simulink library "UAVdesign_net"  (Simulink 7.7)
settings: Solver=ode45  SolverMode=SingleTasking  StartTime=0.0  StopTime=10.0  RelTol=1e-3
undefined symbols (not defined in the file or in its folder): alpha_IERA_IELA_IELA, R_IERA_RA_RA
libraries: UAVdesign_net x75, simulink x13
(part 6 of 8)

== system UAVdesign_net/Subsystem Models/Helicopter Rotor/Rotor Model (IERA)/Rotor Flapping ==
  Parameters : Inport  OutDataTypeStr=Bus: RotorParameters
  Environment : Inport  Port=2  OutDataTypeStr=Bus: Environment
  V_I : Inport  Port=3
  omega_I : Inport  Port=4
  V_dot_I : Inport  Port=5
  omega_dot_I : Inport  Port=6
  V_A : Inport  Port=7
  omega_A : Inport  Port=8
  flap : Inport  Port=9
  cz : Inport  Port=10
  controls : Inport  Port=11
  omega : Inport  Port=12
  Rotor Flapping (Wind-Mast axes) : Stateflow chart  TreatAsAtomicUnit=on
  flap_dot : Outport  PortDimensions=3
  flap_static : Outport  Port=2  PortDimensions=3
  wires:
  Rotor Flapping (Wind-Mast axes)/2(flap_static) -> flap_static/1
  Rotor Flapping (Wind-Mast axes)/1(flap_dot) -> flap_dot/1
  omega/1 -> Rotor Flapping (Wind-Mast axes)/12(omega)
  controls/1 -> Rotor Flapping (Wind-Mast axes)/11(controls)
  cz/1 -> Rotor Flapping (Wind-Mast axes)/10(cz)
  flap/1 -> Rotor Flapping (Wind-Mast axes)/9(flap)
  omega_A/1 -> Rotor Flapping (Wind-Mast axes)/8(oma)
  V_A/1 -> Rotor Flapping (Wind-Mast axes)/7(va)
  omega_dot_I/1 -> Rotor Flapping (Wind-Mast axes)/6(omid)
  V_dot_I/1 -> Rotor Flapping (Wind-Mast axes)/5(vid)
  omega_I/1 -> Rotor Flapping (Wind-Mast axes)/4(omi)
  V_I/1 -> Rotor Flapping (Wind-Mast axes)/3(vi)
  Environment/1 -> Rotor Flapping (Wind-Mast axes)/2(Environment)
  Parameters/1 -> Rotor Flapping (Wind-Mast axes)/1(Parameters)

== system UAVdesign_net/Subsystem Models/Helicopter Rotor/Rotor Model (IERA)/Rotor Forces and Moments ==
  Parameters : Inport  OutDataTypeStr=Bus: RotorParameters
  Environment : Inport  Port=2  OutDataTypeStr=Bus: Environment
  V_A : Inport  Port=3
  omega_A : Inport  Port=4
  omega_dot_I : Inport  Port=5
  flap : Inport  Port=6
  cz : Inport  Port=7
  controls : Inport  Port=8
  omega_rotor : Inport  Port=9
  omega_dot_rotor : Inport  Port=10
  Rotor Forces and Moments (Wind-Mast axes) : Stateflow chart  TreatAsAtomicUnit=on
  FM_A : Outport  PortDimensions=6
  FM_I : Outport  Port=2  PortDimensions=6
  wires:
  Rotor Forces and Moments (Wind-Mast axes)/2(FM_I) -> FM_I/1
  Rotor Forces and Moments (Wind-Mast axes)/1(FM_A) -> FM_A/1
  omega_dot_rotor/1 -> Rotor Forces and Moments (Wind-Mast axes)/10(omegad)
  omega_rotor/1 -> Rotor Forces and Moments (Wind-Mast axes)/9(omega)
  controls/1 -> Rotor Forces and Moments (Wind-Mast axes)/8(controls)
  cz/1 -> Rotor Forces and Moments (Wind-Mast axes)/7(cz)
  flap/1 -> Rotor Forces and Moments (Wind-Mast axes)/6(flap)
  omega_dot_I/1 -> Rotor Forces and Moments (Wind-Mast axes)/5(omid)
  omega_A/1 -> Rotor Forces and Moments (Wind-Mast axes)/4(oma)
  V_A/1 -> Rotor Forces and Moments (Wind-Mast axes)/3(va)
  Environment/1 -> Rotor Forces and Moments (Wind-Mast axes)/2(Environment)
  Parameters/1 -> Rotor Forces and Moments (Wind-Mast axes)/1(Parameters)

== system UAVdesign_net/Subsystem Models/Helicopter Rotor/Rotor Model (IERA)/Rotor Self-Influence ==
  Parameters : Inport  OutDataTypeStr=Bus: RotorParameters
  Environment : Inport  Port=2  OutDataTypeStr=Bus: Environment
  V_A : Inport  Port=3
  omega_A : Inport  Port=4
  FM_A : Inport  Port=5
  Rotor Wash Self-Influence (IERA) : Stateflow chart  TreatAsAtomicUnit=on
  d (k) : Outport  PortDimensions=3
  wires:
  Parameters/1 -> Rotor Wash Self-Influence (IERA)/1(Parameters)
  Rotor Wash Self-Influence (IERA)/1(d) -> d (k)/1
  Environment/1 -> Rotor Wash Self-Influence (IERA)/2(Environment)
  V_A/1 -> Rotor Wash Self-Influence (IERA)/3(va)
  omega_A/1 -> Rotor Wash Self-Influence (IERA)/4(oma)
  FM_A/1 -> Rotor Wash Self-Influence (IERA)/5(FM_A)

== system UAVdesign_net/Subsystem Models/Helicopter Rotor/Rotor Model (IERA)/Rotor Wash Iteration ==
  Parameters : Inport  OutDataTypeStr=Bus: RotorParameters
  V_I : Inport  Port=2
  V_A (k-1) : Inport  Port=3
  omega_A : Inport  Port=4
  bt (k-1) : Inport  Port=5
  eps0 (k-1) : Inport  Port=6
  controls : Inport  Port=7
  omega_rotor : Inport  Port=8
  Rotor Wash Iteration (Wind-Mast axes) : Stateflow chart  TreatAsAtomicUnit=on
  V_A (k) : Outport  PortDimensions=3
  cz (k) : Outport  Port=2  PortDimensions=1
  bt (k) : Outport  Port=3  PortDimensions=1
  eps0 (k) : Outport  Port=4  PortDimensions=1
  wires:
  omega_rotor/1 -> Rotor Wash Iteration (Wind-Mast axes)/8(omega)
  controls/1 -> Rotor Wash Iteration (Wind-Mast axes)/7(controls)
  eps0 (k-1)/1 -> Rotor Wash Iteration (Wind-Mast axes)/6(eps0)
  bt (k-1)/1 -> Rotor Wash Iteration (Wind-Mast axes)/5(bt)
  omega_A/1 -> Rotor Wash Iteration (Wind-Mast axes)/4(oma)
  V_A (k-1)/1 -> Rotor Wash Iteration (Wind-Mast axes)/3(va)
  V_I/1 -> Rotor Wash Iteration (Wind-Mast axes)/2(vi)
  Rotor Wash Iteration (Wind-Mast axes)/4(eps0_new) -> eps0 (k)/1
  Rotor Wash Iteration (Wind-Mast axes)/3(bt_new) -> bt (k)/1
  Rotor Wash Iteration (Wind-Mast axes)/2(cz_new) -> cz (k)/1
  Rotor Wash Iteration (Wind-Mast axes)/1(va_new) -> V_A (k)/1
  Parameters/1 -> Rotor Wash Iteration (Wind-Mast axes)/1(Parameters)

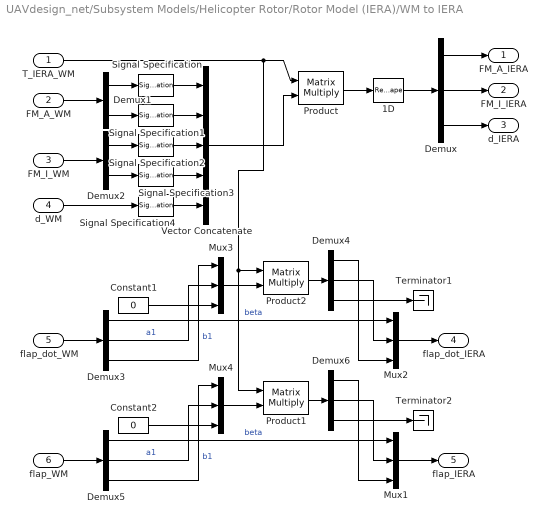
== system UAVdesign_net/Subsystem Models/Helicopter Rotor/Rotor Model (IERA)/WM to IERA ==
  T_IERA_WM : Inport
  FM_A_WM : Inport  Port=2  PortDimensions=6
  FM_I_WM : Inport  Port=3  PortDimensions=6
  d_WM : Inport  Port=4  PortDimensions=3
  flap_dot_WM : Inport  Port=5
  flap_WM : Inport  Port=6
  1D : Reshape
  Constant1 : Constant  Value=0
  Constant2 : Constant  Value=0
  Demux : Demux  Outputs=[6 6 3]
  Demux1 : Demux  Outputs=[3 3]
  Demux2 : Demux  Outputs=[3 3]
  Demux{3..6} (4 alike) : Demux  Outputs=3
  Mux{1..4} (4 alike) : Mux  Inputs=3
  Product : Product  Multiplication=Matrix(*)  RndMeth=Zero
  Product1 : Product  Multiplication=Matrix(*)  RndMeth=Zero
  Product2 : Product  Multiplication=Matrix(*)  RndMeth=Zero
  Signal Specification{,1..4} (5 alike) : SignalSpecification  Dimensions=3
  Terminator1 : Terminator
  Terminator2 : Terminator
  Vector Concatenate : Concatenate  NumInputs=5  Mode=Multidimensional array  ConcatenateDimension=2
  FM_A_IERA : Outport
  FM_I_IERA : Outport  Port=2
  d_IERA : Outport  Port=3
  flap_dot_IERA : Outport  Port=4
  flap_IERA : Outport  Port=5
  wires:
  flap_WM/1 -> Demux5/1
  Mux1/1 -> flap_IERA/1
  Demux5/1 -> Mux1/1  "beta"
  Demux5/2 -> Mux4/2  "a1"
  Demux5/3 -> Mux4/1  "b1"
  Constant2/1 -> Mux4/3
  Mux4/1 -> Product1/2
  Product1/1 -> Demux6/1
  Demux6/1 -> Mux1/3
  Demux6/2 -> Mux1/2
  Demux6/3 -> Terminator2/1
  Demux/2 -> FM_I_IERA/1
  Demux/3 -> d_IERA/1
  FM_I_WM/1 -> Demux2/1
  Demux2/2 -> Signal Specification3/1
  Demux2/1 -> Signal Specification2/1
  d_WM/1 -> Signal Specification4/1
  Demux/1 -> FM_A_IERA/1
  FM_A_WM/1 -> Demux1/1
  Demux1/2 -> Signal Specification1/1
  Demux1/1 -> Signal Specification/1
  1D/1 -> Demux/1
  Product/1 -> 1D/1
  Vector Concatenate/1 -> Product/2
  T_IERA_WM/1 -> Product1/1, Product2/1, Product/1
  flap_dot_WM/1 -> Demux3/1
  Mux2/1 -> flap_dot_IERA/1
  Demux3/1 -> Mux2/1  "beta"
  Demux3/2 -> Mux3/2  "a1"
  Demux3/3 -> Mux3/1  "b1"
  Constant1/1 -> Mux3/3
  Mux3/1 -> Product2/2
  Product2/1 -> Demux4/1
  Demux4/1 -> Mux2/3
  Demux4/2 -> Mux2/2
  Demux4/3 -> Terminator1/1
  Signal Specification/1 -> Vector Concatenate/1
  Signal Specification1/1 -> Vector Concatenate/2
  Signal Specification2/1 -> Vector Concatenate/3
  Signal Specification3/1 -> Vector Concatenate/4
  Signal Specification4/1 -> Vector Concatenate/5

== system UAVdesign_net/Subsystem Models/Helicopter Rotor/Rotor Model (IERA)/Wind-Mast Orientation ==
  V_A : Inport
  Wind Reference Axes : Stateflow chart  TreatAsAtomicUnit=on
  T_WM_IERA : Outport
  T_IERA_WM : Outport  Port=2
  wires:
  V_A/1 -> Wind Reference Axes/1(VA_IERA)
  Wind Reference Axes/1(T_WM_IERA) -> T_WM_IERA/1
  Wind Reference Axes/2(T_IERA_WM) -> T_IERA_WM/1

== system UAVdesign_net/Subsystem Models/Propeller/Rotor Model (IERA)/IERA to WM ==
  T_WM_IERA : Inport
  V_I_IERA : Inport  Port=2
  omega_I_IERA : Inport  Port=3
  V_A_IERA : Inport  Port=4
  omega_A_IERA : Inport  Port=5
  1D : Reshape
  Demux : Demux
  Product : Product  Multiplication=Matrix(*)  RndMeth=Zero
  Vector Concatenate : Concatenate  NumInputs=4  Mode=Multidimensional array  ConcatenateDimension=2
  V_I_WM : Outport
  omega_I_WM : Outport  Port=2
  V_A_WM : Outport  Port=3
  omega_A_WM : Outport  Port=4
  wires:
  Demux/2 -> omega_I_WM/1
  Demux/1 -> V_I_WM/1
  1D/1 -> Demux/1
  Product/1 -> 1D/1
  Vector Concatenate/1 -> Product/2
  omega_I_IERA/1 -> Vector Concatenate/2
  V_I_IERA/1 -> Vector Concatenate/1
  T_WM_IERA/1 -> Product/1
  V_A_IERA/1 -> Vector Concatenate/3
  omega_A_IERA/1 -> Vector Concatenate/4
  Demux/3 -> V_A_WM/1
  Demux/4 -> omega_A_WM/1

== system UAVdesign_net/Subsystem Models/Propeller/Rotor Model (IERA)/Rotor Forces and Moments (Aero) ==
  Parameters : Inport
  Environment : Inport  Port=2
  V_A : Inport  Port=3
  omega_A : Inport  Port=4
  cz : Inport  Port=5
  controls : Inport  Port=6
  omega_rotor : Inport  Port=7
  Rotor Forces and Moments (Wind-Mast axes) : Stateflow chart  TreatAsAtomicUnit=on
  FM_A : Outport  PortDimensions=6
  wires:
  Parameters/1 -> Rotor Forces and Moments (Wind-Mast axes)/1(Parameters)
  Environment/1 -> Rotor Forces and Moments (Wind-Mast axes)/2(Environment)
  V_A/1 -> Rotor Forces and Moments (Wind-Mast axes)/3(va)
  omega_A/1 -> Rotor Forces and Moments (Wind-Mast axes)/4(oma)
  cz/1 -> Rotor Forces and Moments (Wind-Mast axes)/5(cz)
  controls/1 -> Rotor Forces and Moments (Wind-Mast axes)/6(controls)
  omega_rotor/1 -> Rotor Forces and Moments (Wind-Mast axes)/7(omega)
  Rotor Forces and Moments (Wind-Mast axes)/1(FM_A) -> FM_A/1

== system UAVdesign_net/Subsystem Models/Propeller/Rotor Model (IERA)/Rotor Self-Influence ==
  Parameters : Inport
  Environment : Inport  Port=2
  V_A : Inport  Port=3
  omega_A : Inport  Port=4
  FM_A : Inport  Port=5
  Rotor Wash Self-Influence (IERA) : Stateflow chart  TreatAsAtomicUnit=on
  d (k) : Outport  PortDimensions=3
  wires:
  FM_A/1 -> Rotor Wash Self-Influence (IERA)/5(FM_A)
  omega_A/1 -> Rotor Wash Self-Influence (IERA)/4(oma)
  V_A/1 -> Rotor Wash Self-Influence (IERA)/3(va)
  Environment/1 -> Rotor Wash Self-Influence (IERA)/2(Environment)
  Rotor Wash Self-Influence (IERA)/1(d) -> d (k)/1
  Parameters/1 -> Rotor Wash Self-Influence (IERA)/1(Parameters)

== system UAVdesign_net/Subsystem Models/Propeller/Rotor Model (IERA)/Rotor Wash Iteration ==
  Parameters : Inport
  V_I : Inport  Port=2
  V_A (k-1) : Inport  Port=3
  omega_A : Inport  Port=4
  bt (k-1) : Inport  Port=5
  eps0 (k-1) : Inport  Port=6
  controls : Inport  Port=7
  omega_rotor : Inport  Port=8
  Rotor Wash Iteration (Wind-Mast axes) : Stateflow chart  TreatAsAtomicUnit=on
  V_A (k) : Outport  PortDimensions=3
  cz (k) : Outport  Port=2  PortDimensions=1
  bt (k) : Outport  Port=3  PortDimensions=1
  eps0 (k) : Outport  Port=4  PortDimensions=1
  wires:
  Parameters/1 -> Rotor Wash Iteration (Wind-Mast axes)/1(Parameters)
  Rotor Wash Iteration (Wind-Mast axes)/1(va_new) -> V_A (k)/1
  Rotor Wash Iteration (Wind-Mast axes)/2(cz_new) -> cz (k)/1
  Rotor Wash Iteration (Wind-Mast axes)/3(bt_new) -> bt (k)/1
  Rotor Wash Iteration (Wind-Mast axes)/4(eps0_new) -> eps0 (k)/1
  V_I/1 -> Rotor Wash Iteration (Wind-Mast axes)/2(vi)
  V_A (k-1)/1 -> Rotor Wash Iteration (Wind-Mast axes)/3(va)
  omega_A/1 -> Rotor Wash Iteration (Wind-Mast axes)/4(oma)
  bt (k-1)/1 -> Rotor Wash Iteration (Wind-Mast axes)/5(bt)
  eps0 (k-1)/1 -> Rotor Wash Iteration (Wind-Mast axes)/6(eps0)
  controls/1 -> Rotor Wash Iteration (Wind-Mast axes)/7(controls)
  omega_rotor/1 -> Rotor Wash Iteration (Wind-Mast axes)/8(omega)

== system UAVdesign_net/Subsystem Models/Propeller/Rotor Model (IERA)/WM to IERA ==
  T_IERA_WM : Inport
  FM_A_WM : Inport  Port=2  PortDimensions=6
  d_WM : Inport  Port=3  PortDimensions=3
  1D : Reshape
  Demux : Demux  Outputs=[6 3]
  Demux1 : Demux  Outputs=[3 3]
  Product : Product  Multiplication=Matrix(*)  RndMeth=Zero
  Signal Specification : SignalSpecification  Dimensions=3
  Signal Specification1 : SignalSpecification  Dimensions=3
  Signal Specification4 : SignalSpecification  Dimensions=3
  Vector Concatenate : Concatenate  NumInputs=3  Mode=Multidimensional array  ConcatenateDimension=2
  FM_A_IERA : Outport
  d_IERA : Outport  Port=2
  wires:
  Signal Specification4/1 -> Vector Concatenate/3
  Signal Specification1/1 -> Vector Concatenate/2
  Signal Specification/1 -> Vector Concatenate/1
  T_IERA_WM/1 -> Product/1
  Vector Concatenate/1 -> Product/2
  Product/1 -> 1D/1
  1D/1 -> Demux/1
  Demux1/1 -> Signal Specification/1
  Demux1/2 -> Signal Specification1/1
  FM_A_WM/1 -> Demux1/1
  Demux/1 -> FM_A_IERA/1
  d_WM/1 -> Signal Specification4/1
  Demux/2 -> d_IERA/1

== system UAVdesign_net/Subsystem Models/Propeller/Rotor Model (IERA)/Wind-Mast Orientation ==
  V_A : Inport
  Wind Reference Axes : Stateflow chart  TreatAsAtomicUnit=on
  T_WM_IERA : Outport
  T_IERA_WM : Outport  Port=2
  wires:
  Wind Reference Axes/2(T_IERA_WM) -> T_IERA_WM/1
  Wind Reference Axes/1(T_WM_IERA) -> T_WM_IERA/1
  V_A/1 -> Wind Reference Axes/1(VA_IERA)

== system UAVdesign_net/Subsystem Models/Wing/Wing Model (IERA)/Left Wing ==
  Parameters : Inport  OutDataTypeStr=Bus: FinParameters
  Environment : Inport  Port=2  OutDataTypeStr=Bus: Environment
  V_A : Inport  Port=3
  omega_A : Inport  Port=4
  T_WRA_MAC : Inport  Port=5
  T_MAC_WRA : Inport  Port=6
  Left/Right : Inport  Port=7
  Bus Selector : BusSelector  OutputSignals=taper,span,sweep,dihedral
  Half Wing Forces and Moments : Subsystem
      mask Display:
      | port_label('input', 1, 'Parameters', 'texmode', 'on')
      | port_label('input', 2, 'Environment', 'texmode', 'on')
      | port_label('input', 3, 'V_{A|WRA}', 'texmode', 'on')
      | port_label('input', 4, '\omega_{A|WRA}', 'texmode', 'on')
      | 
      | port_label('output', 1, 'FM_{A}', 'texmode', 'on')
  IERA to MAC : Subsystem
      mask Display:
      | port_label('input', 1, 'R_{MAC-IERA|IERA}', 'texmode', 'on')
      | port_label('input', 2, 'V_{A|IERA}', 'texmode', 'on')
      | port_label('input', 3, '\omega_{A|IERA}', 'texmode', 'on')
      | port_label('output', 1, 'V_{A|MAC}', 'texmode', 'on')
      | port_label('output', 2, '\omega_{A|MAC}', 'texmode', 'on')
  MAC to IERA : Subsystem
      mask Display:
      | port_label('input', 1, 'R_{MAC-IERA|IERA}', 'texmode', 'on')
      | port_label('input', 2, 'FM_{MAC}', 'texmode', 'on')
      | port_label('output', 1, 'FM_{IERA}', 'texmode', 'on')
  MAC to WRA (Half Wing) : Subsystem
      mask Display:
      | port_label('input', 1, 'T_{WRA-MAC}', 'texmode', 'on')
      | port_label('input', 2, 'V_{A|MAC}', 'texmode', 'on')
      | port_label('input', 3, '\omega_{A|MAC}', 'texmode', 'on')
      | 
      | port_label('output', 1, 'V_{A|WRA}', 'texmode', 'on')
      | port_label('output', 2, '\omega_{A|WRA}', 'texmode', 'on')
  Mux1 : Mux
  Mux2 : Mux  Inputs=2
  Mux3 : Mux  Inputs=3
  WRA to MAC : Subsystem
      mask Display:
      | port_label('input', 1, 'T_{MAC-WRA}', 'texmode', 'on')
      | port_label('input', 2, 'FM_{A|WRA}', 'texmode', 'on')
      | 
      | port_label('output', 1, 'FM_{A|MAC}', 'texmode', 'on')
  smac : Fcn  Expr=u(2) * (2 * u(1) + 1) / 6 / (u(1) + 1)
  xmac : Fcn  Expr=-sin(u(2)) * cos(-u(3)) * u(1)
  ymac : Fcn  Expr=u(4) * cos(u(2)) * cos(-u(3)) * u(1)
  zmac : Fcn  Expr=sin(-u(3)) * u(1)
  FM_A : Outport
  wires:
  Half Wing Forces and Moments/1(FM_A) -> WRA to MAC/2(FM_A_WM)
  IERA to MAC/1(V_A|MAC) -> MAC to WRA (Half Wing)/2(V_A_MAC)
  IERA to MAC/2(omega_A|MAC) -> MAC to WRA (Half Wing)/3(omega_A_MAC)
  zmac/1 -> Mux3/3
  ymac/1 -> Mux3/2
  xmac/1 -> Mux3/1
  Mux3/1 -> IERA to MAC/1(R_xW-IERA|IERA), MAC to IERA/1(R_MAC_IERA_IERA)
  MAC to WRA (Half Wing)/1(V_A_WRA) -> Half Wing Forces and Moments/3(V_A)
  MAC to WRA (Half Wing)/2(omega_A_WRA) -> Half Wing Forces and Moments/4(omega_A)
  Parameters/1 -> Half Wing Forces and Moments/1(Parameters), Bus Selector/1
  T_WRA_MAC/1 -> MAC to WRA (Half Wing)/1(T_WRA_MAC)
  T_MAC_WRA/1 -> WRA to MAC/1(T_IERA_WM)
  V_A/1 -> IERA to MAC/2(V_A|IERA)
  omega_A/1 -> IERA to MAC/3(omega_A|IERA)
  Mux1/1 -> ymac/1, xmac/1, zmac/1
  Left/Right/1 -> Mux1/4
  smac/1 -> Mux1/1
  Environment/1 -> Half Wing Forces and Moments/2(Environment)
  Bus Selector/1 -> Mux2/1  "<taper>"
  Bus Selector/2 -> Mux2/2  "<span>"
  Mux2/1 -> smac/1
  Bus Selector/3 -> Mux1/2  "<sweep>"
  Bus Selector/4 -> Mux1/3  "<dihedral>"
  WRA to MAC/1(FM_A_IERA) -> MAC to IERA/2(FM_MAC)
  MAC to IERA/1(FM_IERA) -> FM_A/1

== system UAVdesign_net/Subsystem Models/Wing/Wing Model (IERA)/Right Wing ==
  Parameters : Inport  OutDataTypeStr=Bus: FinParameters
  Environment : Inport  Port=2  OutDataTypeStr=Bus: Environment
  V_A : Inport  Port=3
  omega_A : Inport  Port=4
  T_WRA_MAC : Inport  Port=5
  T_MAC_WRA : Inport  Port=6
  Left/Right : Inport  Port=7
  Bus Selector : BusSelector  OutputSignals=taper,span,sweep,dihedral
  Half Wing Forces and Moments : Subsystem
      mask Display:
      | port_label('input', 1, 'Parameters', 'texmode', 'on')
      | port_label('input', 2, 'Environment', 'texmode', 'on')
      | port_label('input', 3, 'V_{A|WRA}', 'texmode', 'on')
      | port_label('input', 4, '\omega_{A|WRA}', 'texmode', 'on')
      | 
      | port_label('output', 1, 'FM_{A}', 'texmode', 'on')
  IERA to MAC : Subsystem
      mask Display:
      | port_label('input', 1, 'R_{MAC-IERA|IERA}', 'texmode', 'on')
      | port_label('input', 2, 'V_{A|IERA}', 'texmode', 'on')
      | port_label('input', 3, '\omega_{A|IERA}', 'texmode', 'on')
      | port_label('output', 1, 'V_{A|MAC}', 'texmode', 'on')
      | port_label('output', 2, '\omega_{A|MAC}', 'texmode', 'on')
  MAC to IERA : Subsystem
      mask Display:
      | port_label('input', 1, 'R_{MAC-IERA|IERA}', 'texmode', 'on')
      | port_label('input', 2, 'FM_{MAC}', 'texmode', 'on')
      | port_label('output', 1, 'FM_{IERA}', 'texmode', 'on')
  MAC to WRA (Half Wing) : Subsystem
      mask Display:
      | port_label('input', 1, 'T_{WRA-MAC}', 'texmode', 'on')
      | port_label('input', 2, 'V_{A|MAC}', 'texmode', 'on')
      | port_label('input', 3, '\omega_{A|MAC}', 'texmode', 'on')
      | 
      | port_label('output', 1, 'V_{A|WRA}', 'texmode', 'on')
      | port_label('output', 2, '\omega_{A|WRA}', 'texmode', 'on')
  Mux1 : Mux
  Mux2 : Mux  Inputs=2
  Mux3 : Mux  Inputs=3
  WRA to MAC : Subsystem
      mask Display:
      | port_label('input', 1, 'T_{MAC-WRA}', 'texmode', 'on')
      | port_label('input', 2, 'FM_{A|WRA}', 'texmode', 'on')
      | 
      | port_label('output', 1, 'FM_{A|MAC}', 'texmode', 'on')
  smac : Fcn  Expr=u(2) * (2 * u(1) + 1) / 6 / (u(1) + 1)
  xmac : Fcn  Expr=-sin(u(2)) * cos(-u(3)) * u(1)
  ymac : Fcn  Expr=u(4) * cos(u(2)) * cos(-u(3)) * u(1)
  zmac : Fcn  Expr=sin(-u(3)) * u(1)
  FM_A : Outport
  wires:
  MAC to IERA/1(FM_IERA) -> FM_A/1
  WRA to MAC/1(FM_A_IERA) -> MAC to IERA/2(FM_MAC)
  Bus Selector/4 -> Mux1/3  "<dihedral>"
  Bus Selector/3 -> Mux1/2  "<sweep>"
  Mux2/1 -> smac/1
  Bus Selector/2 -> Mux2/2  "<span>"
  Bus Selector/1 -> Mux2/1  "<taper>"
  Environment/1 -> Half Wing Forces and Moments/2(Environment)
  smac/1 -> Mux1/1
  Left/Right/1 -> Mux1/4
  Mux1/1 -> zmac/1, xmac/1, ymac/1
  omega_A/1 -> IERA to MAC/3(omega_A|IERA)
  V_A/1 -> IERA to MAC/2(V_A|IERA)
  T_MAC_WRA/1 -> WRA to MAC/1(T_IERA_WM)
  T_WRA_MAC/1 -> MAC to WRA (Half Wing)/1(T_WRA_MAC)
  Parameters/1 -> Bus Selector/1, Half Wing Forces and Moments/1(Parameters)
  MAC to WRA (Half Wing)/2(omega_A_WRA) -> Half Wing Forces and Moments/4(omega_A)
  MAC to WRA (Half Wing)/1(V_A_WRA) -> Half Wing Forces and Moments/3(V_A)
  Mux3/1 -> MAC to IERA/1(R_MAC_IERA_IERA), IERA to MAC/1(R_xW-IERA|IERA)
  xmac/1 -> Mux3/1
  ymac/1 -> Mux3/2
  zmac/1 -> Mux3/3
  IERA to MAC/2(omega_A|MAC) -> MAC to WRA (Half Wing)/3(omega_A_MAC)
  IERA to MAC/1(V_A|MAC) -> MAC to WRA (Half Wing)/2(V_A_MAC)
  Half Wing Forces and Moments/1(FM_A) -> WRA to MAC/2(FM_A_WM)

== system UAVdesign_net/Subsystem Models/Wing/Wing Model (IERA)/Transpose ==
  In : Inport
  Permute Dimensions : PermuteDimensions
  Out : Outport
  wires:
  In/1 -> Permute Dimensions/1
  Permute Dimensions/1 -> Out/1

== system UAVdesign_net/Subsystem Models/Wing/Wing Model (IERA)/Wing Self-Influence ==
  Parameters : Inport  OutDataTypeStr=Bus: FinParameters
  Environment : Inport  Port=2  OutDataTypeStr=Bus: Environment
  V_A : Inport  Port=3
  omega_A : Inport  Port=4
  FM_A : Inport  Port=5
  Wing Wash Self-Influence (IERA : Stateflow chart  TreatAsAtomicUnit=on
  d (k) : Outport
  wires:
  Parameters/1 -> Wing Wash Self-Influence (IERA/1(Parameters)
  Wing Wash Self-Influence (IERA/1(d) -> d (k)/1
  Environment/1 -> Wing Wash Self-Influence (IERA/2(Environment)
  V_A/1 -> Wing Wash Self-Influence (IERA/3(va)
  omega_A/1 -> Wing Wash Self-Influence (IERA/4(oma)
  FM_A/1 -> Wing Wash Self-Influence (IERA/5(FM_A)

== system UAVdesign_net/Utilities/Math/3x3 Cross Product/Subsystem ==
  A : Inport
  B : Inport  Port=2
  Demux : Demux  Outputs=3
  Demux1 : Demux  Outputs=3
  Mux : Mux  Inputs=3
  i x j : Product  SaturateOnIntegerOverflow=on  InputSameDT=on  OutDataTypeStr=Inherit: Same as first input
  j x k : Product  SaturateOnIntegerOverflow=on  InputSameDT=on  OutDataTypeStr=Inherit: Same as first input
  k x i : Product  SaturateOnIntegerOverflow=on  InputSameDT=on  OutDataTypeStr=Inherit: Same as first input
  Out1 : Outport
  wires:
  Mux/1 -> Out1/1
  A/1 -> Demux/1
  B/1 -> Demux1/1
  j x k/1 -> Mux/1
  k x i/1 -> Mux/2
  i x j/1 -> Mux/3
  Demux/1 -> i x j/1
  Demux1/2 -> i x j/2
  Demux1/1 -> k x i/2
  Demux/3 -> k x i/1
  Demux/2 -> j x k/1
  Demux1/3 -> j x k/2

== system UAVdesign_net/Utilities/Math/3x3 Cross Product/Subsystem1 ==
  A : Inport
  B : Inport  Port=2
  Demux : Demux  Outputs=3
  Demux1 : Demux  Outputs=3
  Mux : Mux  Inputs=3
  i x k : Product  SaturateOnIntegerOverflow=on  InputSameDT=on  OutDataTypeStr=Inherit: Same as first input
  j x i : Product  SaturateOnIntegerOverflow=on  InputSameDT=on  OutDataTypeStr=Inherit: Same as first input
  k x j : Product  SaturateOnIntegerOverflow=on  InputSameDT=on  OutDataTypeStr=Inherit: Same as first input
  Out1 : Outport
  wires:
  A/1 -> Demux/1
  B/1 -> Demux1/1
  Demux/3 -> k x j/1
  Demux1/2 -> k x j/2
  Demux/1 -> i x k/1
  Demux1/3 -> i x k/2
  Demux/2 -> j x i/1
  Demux1/1 -> j x i/2
  Mux/1 -> Out1/1
  k x j/1 -> Mux/1
  i x k/1 -> Mux/2
  j x i/1 -> Mux/3

== system UAVdesign_net/Utilities/Math/Adjoint of 3x3 Matrix/C(1,1) ==
  Matrix : Inport
  Product : Product  Inputs=1  SaturateOnIntegerOverflow=on  OutDataTypeStr=Inherit: Same as first input
  Product1 : Product  Inputs=1  SaturateOnIntegerOverflow=on  OutDataTypeStr=Inherit: Same as first input
  Sum : Sum  Inputs=|+-  SaturateOnIntegerOverflow=on
  a(2,2),a(3,3) : Selector  InputPortWidth=9  IndexOptions=Index vector (dialog)  Indices=[5 9]  OutputSizes=1
  a(2,3),a(3,2) : Selector  InputPortWidth=9  IndexOptions=Index vector (dialog)  Indices=[6 8]  OutputSizes=1
  C(1,1) : Outport
  wires:
  a(2,2),a(3,3)/1 -> Product/1
  a(2,3),a(3,2)/1 -> Product1/1
  Product/1 -> Sum/1
  Product1/1 -> Sum/2
  Sum/1 -> C(1,1)/1
  Matrix/1 -> a(2,2),a(3,3)/1, a(2,3),a(3,2)/1

== system UAVdesign_net/Utilities/Math/Adjoint of 3x3 Matrix/C(1,2) ==
  Matrix : Inport
  Product : Product  Inputs=1  SaturateOnIntegerOverflow=on  OutDataTypeStr=Inherit: Same as first input
  Product1 : Product  Inputs=1  SaturateOnIntegerOverflow=on  OutDataTypeStr=Inherit: Same as first input
  Sum : Sum  Inputs=|+-  SaturateOnIntegerOverflow=on
  a(1,2),a(3,3) : Selector  InputPortWidth=9  IndexOptions=Index vector (dialog)  Indices=[4 9]  OutputSizes=1
  a(1,3),a(3,2) : Selector  InputPortWidth=9  IndexOptions=Index vector (dialog)  Indices=[6 7]  OutputSizes=1
  C(1,2) : Outport
  wires:
  Matrix/1 -> a(1,2),a(3,3)/1, a(1,3),a(3,2)/1
  Sum/1 -> C(1,2)/1
  Product1/1 -> Sum/2
  Product/1 -> Sum/1
  a(1,2),a(3,3)/1 -> Product1/1
  a(1,3),a(3,2)/1 -> Product/1

== system UAVdesign_net/Utilities/Math/Adjoint of 3x3 Matrix/C(1,3) ==
  Matrix : Inport
  Product : Product  Inputs=1  SaturateOnIntegerOverflow=on  OutDataTypeStr=Inherit: Same as first input
  Product1 : Product  Inputs=1  SaturateOnIntegerOverflow=on  OutDataTypeStr=Inherit: Same as first input
  Sum : Sum  Inputs=|+-  SaturateOnIntegerOverflow=on
  a(1,2),a(2,3) : Selector  InputPortWidth=9  IndexOptions=Index vector (dialog)  Indices=[4 8]  OutputSizes=1
  a(1,3),a(2,2) : Selector  InputPortWidth=9  IndexOptions=Index vector (dialog)  Indices=[5 7]  OutputSizes=1
  C(1,3) : Outport
  wires:
  a(1,2),a(2,3)/1 -> Product/1
  a(1,3),a(2,2)/1 -> Product1/1
  Product/1 -> Sum/1
  Product1/1 -> Sum/2
  Sum/1 -> C(1,3)/1
  Matrix/1 -> a(1,3),a(2,2)/1, a(1,2),a(2,3)/1

== system UAVdesign_net/Utilities/Math/Adjoint of 3x3 Matrix/C(2,1) ==
  Matrix : Inport
  Product : Product  Inputs=1  SaturateOnIntegerOverflow=on  OutDataTypeStr=Inherit: Same as first input
  Product1 : Product  Inputs=1  SaturateOnIntegerOverflow=on  OutDataTypeStr=Inherit: Same as first input
  Sum : Sum  Inputs=|+-  SaturateOnIntegerOverflow=on
  a(2,1),a(3,3) : Selector  InputPortWidth=9  IndexOptions=Index vector (dialog)  Indices=[2 9]  OutputSizes=1
  a(3,1),a(2,3) : Selector  InputPortWidth=9  IndexOptions=Index vector (dialog)  Indices=[3 8]  OutputSizes=1
  C(2,1) : Outport
  wires:
  Matrix/1 -> a(2,1),a(3,3)/1, a(3,1),a(2,3)/1
  Sum/1 -> C(2,1)/1
  Product1/1 -> Sum/2
  Product/1 -> Sum/1
  a(2,1),a(3,3)/1 -> Product1/1
  a(3,1),a(2,3)/1 -> Product/1

== system UAVdesign_net/Utilities/Math/Adjoint of 3x3 Matrix/C(2,2) ==
  Matrix : Inport
  Product : Product  Inputs=1  SaturateOnIntegerOverflow=on  OutDataTypeStr=Inherit: Same as first input
  Product1 : Product  Inputs=1  SaturateOnIntegerOverflow=on  OutDataTypeStr=Inherit: Same as first input
  Sum : Sum  Inputs=|+-  SaturateOnIntegerOverflow=on
  a(1,1),a(3,3) : Selector  InputPortWidth=9  IndexOptions=Index vector (dialog)  Indices=[1 9]  OutputSizes=1
  a(1,3),a(3,1) : Selector  InputPortWidth=9  IndexOptions=Index vector (dialog)  Indices=[3 7]  OutputSizes=1
  C(2,2) : Outport
  wires:
  a(1,1),a(3,3)/1 -> Product/1
  a(1,3),a(3,1)/1 -> Product1/1
  Product/1 -> Sum/1
  Product1/1 -> Sum/2
  Sum/1 -> C(2,2)/1
  Matrix/1 -> a(1,1),a(3,3)/1, a(1,3),a(3,1)/1

== system UAVdesign_net/Utilities/Math/Adjoint of 3x3 Matrix/C(2,3) ==
  Matrix : Inport
  Product : Product  Inputs=1  SaturateOnIntegerOverflow=on  OutDataTypeStr=Inherit: Same as first input
  Product1 : Product  Inputs=1  SaturateOnIntegerOverflow=on  OutDataTypeStr=Inherit: Same as first input
  Sum : Sum  Inputs=|+-  SaturateOnIntegerOverflow=on
  a(1,1),a(2,3) : Selector  InputPortWidth=9  IndexOptions=Index vector (dialog)  Indices=[1 8]  OutputSizes=1
  a(1,3),a(2,1) : Selector  InputPortWidth=9  IndexOptions=Index vector (dialog)  Indices=[2 7]  OutputSizes=1
  C(2,3) : Outport
  wires:
  Matrix/1 -> a(1,1),a(2,3)/1, a(1,3),a(2,1)/1
  Sum/1 -> C(2,3)/1
  Product1/1 -> Sum/2
  Product/1 -> Sum/1
  a(1,1),a(2,3)/1 -> Product1/1
  a(1,3),a(2,1)/1 -> Product/1

== system UAVdesign_net/Utilities/Math/Adjoint of 3x3 Matrix/C(3,1) ==
  Matrix : Inport
  Product : Product  Inputs=1  SaturateOnIntegerOverflow=on  OutDataTypeStr=Inherit: Same as first input
  Product1 : Product  Inputs=1  SaturateOnIntegerOverflow=on  OutDataTypeStr=Inherit: Same as first input
  Sum : Sum  Inputs=|+-  SaturateOnIntegerOverflow=on
  a(3,1),a(2,2) : Selector  InputPortWidth=9  IndexOptions=Index vector (dialog)  Indices=[3 5]  OutputSizes=1
  a(3,2),a(2,1) : Selector  InputPortWidth=9  IndexOptions=Index vector (dialog)  Indices=[2 6]  OutputSizes=1
  C(3,1) : Outport
  wires:
  a(3,2),a(2,1)/1 -> Product/1
  a(3,1),a(2,2)/1 -> Product1/1
  Product/1 -> Sum/1
  Product1/1 -> Sum/2
  Sum/1 -> C(3,1)/1
  Matrix/1 -> a(3,2),a(2,1)/1, a(3,1),a(2,2)/1

== system UAVdesign_net/Utilities/Math/Adjoint of 3x3 Matrix/C(3,2) ==
  Matrix : Inport
  Product : Product  Inputs=1  SaturateOnIntegerOverflow=on  OutDataTypeStr=Inherit: Same as first input
  Product1 : Product  Inputs=1  SaturateOnIntegerOverflow=on  OutDataTypeStr=Inherit: Same as first input
  Sum : Sum  Inputs=|+-  SaturateOnIntegerOverflow=on
  a(1,1),a(3,2) : Selector  InputPortWidth=9  IndexOptions=Index vector (dialog)  Indices=[1 6]  OutputSizes=1
  a(1,2),a(3,1) : Selector  InputPortWidth=9  IndexOptions=Index vector (dialog)  Indices=[3 4]  OutputSizes=1
  C(3,2) : Outport
  wires:
  Matrix/1 -> a(1,1),a(3,2)/1, a(1,2),a(3,1)/1
  Sum/1 -> C(3,2)/1
  Product1/1 -> Sum/2
  Product/1 -> Sum/1
  a(1,1),a(3,2)/1 -> Product1/1
  a(1,2),a(3,1)/1 -> Product/1

== system UAVdesign_net/Utilities/Math/Adjoint of 3x3 Matrix/C(3,3) ==
  Matrix : Inport
  Product : Product  Inputs=1  SaturateOnIntegerOverflow=on  OutDataTypeStr=Inherit: Same as first input
  Product1 : Product  Inputs=1  SaturateOnIntegerOverflow=on  OutDataTypeStr=Inherit: Same as first input
  Sum : Sum  Inputs=|+-  SaturateOnIntegerOverflow=on
  a(1,1),a(2,2) : Selector  InputPortWidth=9  IndexOptions=Index vector (dialog)  Indices=[1 5]  OutputSizes=1
  a(1,2),a(2,1) : Selector  InputPortWidth=9  IndexOptions=Index vector (dialog)  Indices=[2 4]  OutputSizes=1
  C(3,3) : Outport
  wires:
  Matrix/1 -> a(1,2),a(2,1)/1, a(1,1),a(2,2)/1
  Sum/1 -> C(3,3)/1
  Product1/1 -> Sum/2
  Product/1 -> Sum/1
  a(1,2),a(2,1)/1 -> Product1/1
  a(1,1),a(2,2)/1 -> Product/1

== system UAVdesign_net/Utilities/Math/Quaternion Division/q0 ==
  q : Inport
  r : Inport  Port=2
  Demux : Demux
  Demux1 : Demux
  Product{,1..3} (4 alike) : Product  RndMeth=Zero
  Sum : Sum  Inputs=4
  q0 : Outport
  wires:
  Product2/1 -> Sum/3
  Sum/1 -> q0/1
  Product3/1 -> Sum/4
  Product1/1 -> Sum/2
  Product/1 -> Sum/1
  Demux/4 -> Product3/1
  Demux1/4 -> Product3/2
  Demux1/3 -> Product2/2
  Demux/3 -> Product2/1
  Demux1/2 -> Product1/2
  Demux/2 -> Product1/1
  Demux1/1 -> Product/2
  Demux/1 -> Product/1
  r/1 -> Demux1/1
  q/1 -> Demux/1

== system UAVdesign_net/Utilities/Math/Quaternion Division/q1 ==
  q : Inport
  r : Inport  Port=2
  Demux : Demux
  Demux1 : Demux
  Product{,1..3} (4 alike) : Product  RndMeth=Zero
  Sum : Sum  Inputs=-++-
  q1 : Outport
  wires:
  Demux1/3 -> Product3/2
  Demux1/4 -> Product2/2
  Demux1/1 -> Product1/2
  Demux1/2 -> Product/2
  q/1 -> Demux/1
  r/1 -> Demux1/1
  Demux/1 -> Product/1
  Demux/2 -> Product1/1
  Demux/3 -> Product2/1
  Demux/4 -> Product3/1
  Product/1 -> Sum/1
  Product1/1 -> Sum/2
  Product3/1 -> Sum/4
  Sum/1 -> q1/1
  Product2/1 -> Sum/3

== system UAVdesign_net/Utilities/Math/Quaternion Division/q2 ==
  q : Inport
  r : Inport  Port=2
  Demux : Demux
  Demux1 : Demux
  Product{,1..3} (4 alike) : Product  RndMeth=Zero
  Sum : Sum  Inputs=--++
  q2 : Outport
  wires:
  Demux1/2 -> Product3/2
  Demux1/1 -> Product2/2
  Demux1/4 -> Product1/2
  Demux1/3 -> Product/2
  Product2/1 -> Sum/3
  Sum/1 -> q2/1
  Product3/1 -> Sum/4
  Product1/1 -> Sum/2
  Product/1 -> Sum/1
  Demux/4 -> Product3/1
  Demux/3 -> Product2/1
  Demux/2 -> Product1/1
  Demux/1 -> Product/1
  r/1 -> Demux1/1
  q/1 -> Demux/1

== system UAVdesign_net/Utilities/Math/Quaternion Division/q3 ==
  q : Inport
  r : Inport  Port=2
  Demux : Demux
  Demux1 : Demux
  Product{,1..3} (4 alike) : Product  RndMeth=Zero
  Sum : Sum  Inputs=-+-+
  q3 : Outport
  wires:
  Demux1/4 -> Product/2
  Demux1/3 -> Product1/2
  Demux1/1 -> Product3/2
  Demux1/2 -> Product2/2
  q/1 -> Demux/1
  r/1 -> Demux1/1
  Demux/1 -> Product/1
  Demux/2 -> Product1/1
  Demux/3 -> Product2/1
  Demux/4 -> Product3/1
  Product/1 -> Sum/1
  Product1/1 -> Sum/2
  Product3/1 -> Sum/4
  Sum/1 -> q3/1
  Product2/1 -> Sum/3

== system UAVdesign_net/Utilities/Math/Quaternion Multiplication/q0 ==
  q : Inport
  r : Inport  Port=2
  Demux : Demux
  Demux1 : Demux
  Product{,1..3} (4 alike) : Product  RndMeth=Zero
  Sum : Sum  Inputs=+---
  q0 : Outport
  wires:
  q/1 -> Demux/1
  r/1 -> Demux1/1
  Demux/1 -> Product/1
  Demux1/1 -> Product/2
  Demux/2 -> Product1/1
  Demux1/2 -> Product1/2
  Demux/3 -> Product2/1
  Demux1/3 -> Product2/2
  Demux1/4 -> Product3/2
  Demux/4 -> Product3/1
  Product/1 -> Sum/1
  Product1/1 -> Sum/2
  Product3/1 -> Sum/4
  Sum/1 -> q0/1
  Product2/1 -> Sum/3

== system UAVdesign_net/Utilities/Math/Quaternion Multiplication/q1 ==
  q : Inport
  r : Inport  Port=2
  Demux : Demux
  Demux1 : Demux
  Product{,1..3} (4 alike) : Product  RndMeth=Zero
  Sum : Sum  Inputs=+++-
  q1 : Outport
  wires:
  Product2/1 -> Sum/3
  Sum/1 -> q1/1
  Product3/1 -> Sum/4
  Product1/1 -> Sum/2
  Product/1 -> Sum/1
  Demux/4 -> Product3/1
  Demux/3 -> Product2/1
  Demux/2 -> Product1/1
  Demux/1 -> Product/1
  r/1 -> Demux1/1
  q/1 -> Demux/1
  Demux1/2 -> Product/2
  Demux1/1 -> Product1/2
  Demux1/4 -> Product2/2
  Demux1/3 -> Product3/2

== system UAVdesign_net/Utilities/Math/Quaternion Multiplication/q2 ==
  q : Inport
  r : Inport  Port=2
  Demux : Demux
  Demux1 : Demux
  Product{,1..3} (4 alike) : Product  RndMeth=Zero
  Sum : Sum  Inputs=+-++
  q2 : Outport
  wires:
  q/1 -> Demux/1
  r/1 -> Demux1/1
  Demux/1 -> Product/1
  Demux/2 -> Product1/1
  Demux/3 -> Product2/1
  Demux/4 -> Product3/1
  Product/1 -> Sum/1
  Product1/1 -> Sum/2
  Product3/1 -> Sum/4
  Sum/1 -> q2/1
  Product2/1 -> Sum/3
  Demux1/3 -> Product/2
  Demux1/4 -> Product1/2
  Demux1/1 -> Product2/2
  Demux1/2 -> Product3/2

== system UAVdesign_net/Utilities/Math/Quaternion Multiplication/q3 ==
  q : Inport
  r : Inport  Port=2
  Demux : Demux
  Demux1 : Demux
  Product{,1..3} (4 alike) : Product  RndMeth=Zero
  Sum : Sum  Inputs=++-+
  q3 : Outport
  wires:
  Product2/1 -> Sum/3
  Sum/1 -> q3/1
  Product3/1 -> Sum/4
  Product1/1 -> Sum/2
  Product/1 -> Sum/1
  Demux/4 -> Product3/1
  Demux/3 -> Product2/1
  Demux/2 -> Product1/1
  Demux/1 -> Product/1
  r/1 -> Demux1/1
  q/1 -> Demux/1
  Demux1/2 -> Product2/2
  Demux1/1 -> Product3/2
  Demux1/3 -> Product1/2
  Demux1/4 -> Product/2

== system UAVdesign_net/Utilities/Math/Quaternion Rotation (B<E)/V1 ==
  q : Inport
  vec : Inport  Port=2
  Constant : Constant  Value=0.5
  Demux : Demux
  Demux1 : Demux  Outputs=3
  Demux2 : Demux
  Demux3 : Demux
  Gain : Gain  Gain=2
  Gain1 : Gain  Gain=2
  Gain2 : Gain  Gain=2
  Product{,1..8} (9 alike) : Product  RndMeth=Zero
  Sum : Sum  Inputs=3
  Sum1 : Sum  Inputs=+|+
  Sum2 : Sum  Inputs=-+|
  Sum3 : Sum  Inputs=--+
  Terminator1 : Terminator
  Terminator2 : Terminator
  V1 : Outport
  wires:
  Demux/3 -> Product/2
  Demux/4 -> Product1/2
  Sum/1 -> V1/1
  Product1/1 -> Sum1/2
  Product/1 -> Sum1/1
  vec/1 -> Demux1/1
  q/1 -> Demux/1, Demux2/1, Demux3/1
  Demux/2 -> Product/1
  Demux/1 -> Product1/1
  Sum1/1 -> Gain/1
  Gain/1 -> Product4/1
  Product3/1 -> Sum2/2
  Product2/1 -> Sum2/1
  Sum2/1 -> Gain1/1
  Demux2/1 -> Product2/1
  Demux2/3 -> Product2/2
  Demux2/4 -> Product3/2
  Gain1/1 -> Product5/1
  Product6/1 -> Sum3/1
  Product7/1 -> Sum3/2
  Sum3/1 -> Gain2/1
  Gain2/1 -> Product8/2
  Demux3/4 -> Product7/1, Product7/2
  Demux3/1 -> Terminator1/1
  Constant/1 -> Sum3/3
  Product4/1 -> Sum/2
  Demux1/1 -> Product8/1
  Demux1/2 -> Product4/2
  Demux3/3 -> Product6/2, Product6/1
  Demux3/2 -> Terminator2/1
  Product8/1 -> Sum/1
  Demux2/2 -> Product3/1
  Demux1/3 -> Product5/2
  Product5/1 -> Sum/3

== system UAVdesign_net/Utilities/Math/Quaternion Rotation (B<E)/V2 ==
  q : Inport
  vec : Inport  Port=2
  Constant : Constant  Value=0.5
  Demux : Demux
  Demux1 : Demux  Outputs=3
  Demux2 : Demux
  Demux3 : Demux
  Gain : Gain  Gain=2
  Gain1 : Gain  Gain=2
  Gain2 : Gain  Gain=2
  Product{,1..8} (9 alike) : Product  RndMeth=Zero
  Sum : Sum  Inputs=3
  Sum1 : Sum  Inputs=+|-
  Sum2 : Sum  Inputs=++|
  Sum3 : Sum  Inputs=--+
  Terminator1 : Terminator
  Terminator2 : Terminator
  V2 : Outport
  wires:
  Constant/1 -> Sum3/3
  Demux3/1 -> Terminator1/1
  Demux3/4 -> Product7/2, Product7/1
  Gain2/1 -> Product8/1
  Sum3/1 -> Gain2/1
  Product7/1 -> Sum3/2
  Product6/1 -> Sum3/1
  Demux3/2 -> Product6/1, Product6/2
  Product4/1 -> Sum/1
  Gain1/1 -> Product5/1
  Demux2/4 -> Product3/2
  Demux2/3 -> Product3/1
  Demux2/2 -> Product2/2
  Demux2/1 -> Product2/1
  Sum2/1 -> Gain1/1
  Product2/1 -> Sum2/1
  Product3/1 -> Sum2/2
  Gain/1 -> Product4/2
  Sum1/1 -> Gain/1
  Demux/1 -> Product1/1
  Demux/2 -> Product/1
  q/1 -> Demux3/1, Demux2/1, Demux/1
  vec/1 -> Demux1/1
  Product/1 -> Sum1/1
  Product1/1 -> Sum1/2
  Sum/1 -> V2/1
  Demux/4 -> Product1/2
  Demux/3 -> Product/2
  Demux1/1 -> Product4/1
  Demux3/3 -> Terminator2/1
  Demux1/2 -> Product8/2
  Product8/1 -> Sum/2
  Product5/1 -> Sum/3
  Demux1/3 -> Product5/2

== system UAVdesign_net/Utilities/Math/Quaternion Rotation (B<E)/V3 ==
  q : Inport
  vec : Inport  Port=2
  Constant : Constant  Value=0.5
  Demux : Demux
  Demux1 : Demux  Outputs=3
  Demux2 : Demux
  Demux3 : Demux
  Gain : Gain  Gain=2
  Gain1 : Gain  Gain=2
  Gain2 : Gain  Gain=2
  Product{,1..8} (9 alike) : Product  RndMeth=Zero
  Sum : Sum  Inputs=3
  Sum1 : Sum  Inputs=+|+
  Sum2 : Sum  Inputs=-+|
  Sum3 : Sum  Inputs=--+
  Terminator : Terminator
  Terminator1 : Terminator
  V3 : Outport
  wires:
  Sum/1 -> V3/1
  Product1/1 -> Sum1/2
  Product/1 -> Sum1/1
  vec/1 -> Demux1/1
  q/1 -> Demux/1, Demux2/1, Demux3/1
  Demux/4 -> Product/2
  Demux/2 -> Product/1
  Demux/1 -> Product1/1
  Demux/3 -> Product1/2
  Sum1/1 -> Gain/1
  Gain/1 -> Product4/2
  Demux1/1 -> Product4/1
  Product3/1 -> Sum2/2
  Product2/1 -> Sum2/1
  Sum2/1 -> Gain1/1
  Demux2/1 -> Product2/1
  Demux2/2 -> Product2/2
  Demux2/3 -> Product3/1
  Demux2/4 -> Product3/2
  Gain1/1 -> Product5/1
  Demux1/2 -> Product5/2
  Product5/1 -> Sum/2
  Product4/1 -> Sum/1
  Demux3/2 -> Product6/2, Product6/1
  Demux3/3 -> Product7/1, Product7/2
  Product6/1 -> Sum3/1
  Product7/1 -> Sum3/2
  Sum3/1 -> Gain2/1
  Gain2/1 -> Product8/1
  Demux3/4 -> Terminator/1
  Demux3/1 -> Terminator1/1
  Constant/1 -> Sum3/3
  Demux1/3 -> Product8/2
  Product8/1 -> Sum/3

== system UAVdesign_net/Utilities/Math/Quaternion Rotation (E<B)/V1 ==
  q : Inport
  vec : Inport  Port=2
  Constant : Constant  Value=0.5
  Demux : Demux
  Demux1 : Demux  Outputs=3
  Demux2 : Demux
  Demux3 : Demux
  Gain : Gain  Gain=2
  Gain1 : Gain  Gain=2
  Gain2 : Gain  Gain=2
  Product{,1..8} (9 alike) : Product  RndMeth=Zero
  Sum : Sum  Inputs=3
  Sum1 : Sum  Inputs=+|+
  Sum2 : Sum  Inputs=-+|
  Sum3 : Sum  Inputs=--+
  Terminator1 : Terminator
  Terminator2 : Terminator
  V1 : Outport
  wires:
  Product5/1 -> Sum/3
  Demux1/3 -> Product5/2
  Demux2/2 -> Product3/1
  Product8/1 -> Sum/1
  Demux3/2 -> Terminator2/1
  Demux3/3 -> Product6/1, Product6/2
  Demux1/2 -> Product4/2
  Demux1/1 -> Product8/1
  Product4/1 -> Sum/2
  Constant/1 -> Sum3/3
  Demux3/1 -> Terminator1/1
  Demux3/4 -> Product7/2, Product7/1
  Gain2/1 -> Product8/2
  Sum3/1 -> Gain2/1
  Product7/1 -> Sum3/2
  Product6/1 -> Sum3/1
  Gain1/1 -> Product5/1
  Demux2/4 -> Product3/2
  Demux2/3 -> Product2/2
  Demux2/1 -> Product2/1
  Sum2/1 -> Gain1/1
  Product2/1 -> Sum2/1
  Product3/1 -> Sum2/2
  Gain/1 -> Product4/1
  Sum1/1 -> Gain/1
  Demux/1 -> Product1/1
  Demux/2 -> Product/1
  q/1 -> Demux3/1, Demux2/1, Demux/1
  vec/1 -> Demux1/1
  Product/1 -> Sum1/1
  Product1/1 -> Sum1/2
  Sum/1 -> V1/1
  Demux/4 -> Product1/2
  Demux/3 -> Product/2

== system UAVdesign_net/Utilities/Math/Quaternion Rotation (E<B)/V2 ==
  q : Inport
  vec : Inport  Port=2
  Constant : Constant  Value=0.5
  Demux : Demux
  Demux1 : Demux  Outputs=3
  Demux2 : Demux
  Demux3 : Demux
  Gain : Gain  Gain=2
  Gain1 : Gain  Gain=2
  Gain2 : Gain  Gain=2
  Product{,1..8} (9 alike) : Product  RndMeth=Zero
  Sum : Sum  Inputs=3
  Sum1 : Sum  Inputs=+|-
  Sum2 : Sum  Inputs=++|
  Sum3 : Sum  Inputs=--+
  Terminator1 : Terminator
  Terminator2 : Terminator
  V2 : Outport
  wires:
  Demux1/3 -> Product5/2
  Product5/1 -> Sum/3
  Product8/1 -> Sum/2
  Demux1/2 -> Product8/2
  Demux3/3 -> Terminator2/1
  Demux1/1 -> Product4/1
  Demux/3 -> Product/2
  Demux/4 -> Product1/2
  Sum/1 -> V2/1
  Product1/1 -> Sum1/2
  Product/1 -> Sum1/1
  vec/1 -> Demux1/1
  q/1 -> Demux/1, Demux2/1, Demux3/1
  Demux/2 -> Product/1
  Demux/1 -> Product1/1
  Sum1/1 -> Gain/1
  Gain/1 -> Product4/2
  Product3/1 -> Sum2/2
  Product2/1 -> Sum2/1
  Sum2/1 -> Gain1/1
  Demux2/1 -> Product2/1
  Demux2/2 -> Product2/2
  Demux2/3 -> Product3/1
  Demux2/4 -> Product3/2
  Gain1/1 -> Product5/1
  Product4/1 -> Sum/1
  Demux3/2 -> Product6/2, Product6/1
  Product6/1 -> Sum3/1
  Product7/1 -> Sum3/2
  Sum3/1 -> Gain2/1
  Gain2/1 -> Product8/1
  Demux3/4 -> Product7/1, Product7/2
  Demux3/1 -> Terminator1/1
  Constant/1 -> Sum3/3

== system UAVdesign_net/Utilities/Math/Quaternion Rotation (E<B)/V3 ==
  q : Inport
  vec : Inport  Port=2
  Constant : Constant  Value=0.5
  Demux : Demux
  Demux1 : Demux  Outputs=3
  Demux2 : Demux
  Demux3 : Demux
  Gain : Gain  Gain=2
  Gain1 : Gain  Gain=2
  Gain2 : Gain  Gain=2
  Product{,1..8} (9 alike) : Product  RndMeth=Zero
  Sum : Sum  Inputs=3
  Sum1 : Sum  Inputs=+|+
  Sum2 : Sum  Inputs=-+|
  Sum3 : Sum  Inputs=--+
  Terminator : Terminator
  Terminator1 : Terminator
  V3 : Outport
  wires:
  Product8/1 -> Sum/3
  Demux1/3 -> Product8/2
  Constant/1 -> Sum3/3
  Demux3/1 -> Terminator1/1
  Demux3/4 -> Terminator/1
  Gain2/1 -> Product8/1
  Sum3/1 -> Gain2/1
  Product7/1 -> Sum3/2
  Product6/1 -> Sum3/1
  Demux3/3 -> Product7/2, Product7/1
  Demux3/2 -> Product6/1, Product6/2
  Product4/1 -> Sum/1
  Product5/1 -> Sum/2
  Demux1/2 -> Product5/2
  Gain1/1 -> Product5/1
  Demux2/4 -> Product3/2
  Demux2/3 -> Product3/1
  Demux2/2 -> Product2/2
  Demux2/1 -> Product2/1
  Sum2/1 -> Gain1/1
  Product2/1 -> Sum2/1
  Product3/1 -> Sum2/2
  Demux1/1 -> Product4/1
  Gain/1 -> Product4/2
  Sum1/1 -> Gain/1
  Demux/3 -> Product1/2
  Demux/1 -> Product1/1
  Demux/2 -> Product/1
  Demux/4 -> Product/2
  q/1 -> Demux3/1, Demux2/1, Demux/1
  vec/1 -> Demux1/1
  Product/1 -> Sum1/1
  Product1/1 -> Sum1/2
  Sum/1 -> V3/1

== system UAVdesign_net/Vehicle Models/Helicopter Model/RA to IELA CG computation/RA to IELA ==
  Geometry : Inport  OutDataTypeStr=Bus: GeometryParameters
  CG_RA_RA : Inport  Port=2
  Bus Selector : BusSelector  OutputSignals=R_IERA_RA_RA,alpha_IERA_IELA_IELA,m,I_IERA
  Dot Product : simulink/Math Operations/Dot Product  InputSameDT=on  OutDataType=sfix(16)  OutScaling=2^-10  DoSatur=off
  Identity matrix : Constant  Value=[1 0 0; 0 1 0; 0 0 1]
  Product : Product  RndMeth=Zero
  Product1 : Product  RndMeth=Zero
  Product2 : Product  Multiplication=Matrix(*)  RndMeth=Zero
  Product3 : Product  RndMeth=Zero
  RA to IELA1 : Subsystem
  Reshape : Reshape  OutputDimensionality=Column vector (2-D)
  Reshape1 : Reshape  OutputDimensionality=Row vector (2-D)
  Rotate to IELA : Product  Inputs=3  Multiplication=Matrix(*)  RndMeth=Zero
  Rotation Matrix from IELA to IERA : UAVdesign_net/Utilities/Axes/Euler Rotation Matrix from Earth to Body  SystemSampleTime=-1
  Sum : Sum  Inputs=-+|
  Sum1 : Sum  Inputs=+|+
  Sum2 : Sum  Inputs=|+-
  Transpose : Subsystem
      mask Display: disp('A^T', 'texmode', 'on')
  R_IELA_B_B : Outport
  alpha_IERA_IELA : Outport  Port=2
  T_IERA_IELA : Outport  Port=3
  T_IELA_IERA : Outport  Port=4
  mass_distance : Outport  Port=5
  m : Outport  Port=6
  I_CG : Outport  Port=7
  wires:
  Bus Selector/1 -> Product/1, Sum/2  "<R_IERA_RA_RA>"
  Bus Selector/2 -> alpha_IERA_IELA/1, Rotation Matrix from IELA to IERA/1  "<alpha_IERA_IELA_IELA>"
  Bus Selector/3 -> Product/2, Product1/1, m/1  "<m>"
  Sum/1 -> RA to IELA1/1(RA)
  Product1/1 -> Sum1/2
  Reshape/1 -> Product2/1
  Reshape1/1 -> Product2/2
  Dot Product/1 -> Product3/2
  Identity matrix/1 -> Product3/1
  Product3/1 -> Sum2/1
  Product2/1 -> Sum2/2
  Sum2/1 -> Product1/2
  Geometry/1 -> Bus Selector/1
  Product/1 -> mass_distance/1
  Sum1/1 -> I_CG/1
  CG_RA_RA/1 -> Sum/1
  RA to IELA1/1(IELA) -> Dot Product/1, Dot Product/2, Reshape1/1, Reshape/1, R_IELA_B_B/1
  Rotation Matrix from IELA to IERA/1 -> Transpose/1(In), T_IERA_IELA/1, Rotate to IELA/1
  Transpose/1(Out) -> T_IELA_IERA/1, Rotate to IELA/3
  Rotate to IELA/1 -> Sum1/1
  Bus Selector/4 -> Rotate to IELA/2  "<I_IERA>"

== system UAVdesign_net/Vehicle Models/Helicopter Model/RA to IELA CG computation/RA to IELA 2 ==
  Geometry : Inport  OutDataTypeStr=Bus: GeometryParameters
  CG_RA_RA : Inport  Port=2
  Bus Selector : BusSelector  OutputSignals=R_IERA_RA_RA,alpha_IERA_IELA_IELA,m,I_IERA
  Dot Product : simulink/Math Operations/Dot Product  InputSameDT=on  OutDataType=sfix(16)  OutScaling=2^-10  DoSatur=off
  Identity matrix : Constant  Value=[1 0 0; 0 1 0; 0 0 1]
  Product : Product  RndMeth=Zero
  Product1 : Product  RndMeth=Zero
  Product2 : Product  Multiplication=Matrix(*)  RndMeth=Zero
  Product3 : Product  RndMeth=Zero
  RA to IELA1 : Subsystem
  Reshape : Reshape  OutputDimensionality=Column vector (2-D)
  Reshape1 : Reshape  OutputDimensionality=Row vector (2-D)
  Rotate to IELA : Product  Inputs=3  Multiplication=Matrix(*)  RndMeth=Zero
  Rotation Matrix from IELA to IERA : UAVdesign_net/Utilities/Axes/Euler Rotation Matrix from Earth to Body  SystemSampleTime=-1
  Sum : Sum  Inputs=-+|
  Sum1 : Sum  Inputs=+|+
  Sum2 : Sum  Inputs=|+-
  Transpose : Subsystem
      mask Display: disp('A^T', 'texmode', 'on')
  R_IELA_B_B : Outport
  alpha_IERA_IELA : Outport  Port=2
  T_IERA_IELA : Outport  Port=3
  T_IELA_IERA : Outport  Port=4
  mass_distance : Outport  Port=5
  m : Outport  Port=6
  I_CG : Outport  Port=7
  wires:
  Bus Selector/4 -> Rotate to IELA/2  "<I_IERA>"
  Rotate to IELA/1 -> Sum1/1
  Transpose/1(Out) -> Rotate to IELA/3, T_IELA_IERA/1
  Rotation Matrix from IELA to IERA/1 -> Rotate to IELA/1, T_IERA_IELA/1, Transpose/1(In)
  RA to IELA1/1(IELA) -> R_IELA_B_B/1, Reshape/1, Reshape1/1, Dot Product/2, Dot Product/1
  CG_RA_RA/1 -> Sum/1
  Sum1/1 -> I_CG/1
  Product/1 -> mass_distance/1
  Geometry/1 -> Bus Selector/1
  Sum2/1 -> Product1/2
  Product2/1 -> Sum2/2
  Product3/1 -> Sum2/1
  Identity matrix/1 -> Product3/1
  Dot Product/1 -> Product3/2
  Reshape1/1 -> Product2/2
  Reshape/1 -> Product2/1
  Product1/1 -> Sum1/2
  Sum/1 -> RA to IELA1/1(RA)
  Bus Selector/3 -> m/1, Product1/1, Product/2  "<m>"
  Bus Selector/2 -> Rotation Matrix from IELA to IERA/1, alpha_IERA_IELA/1  "<alpha_IERA_IELA_IELA>"
  Bus Selector/1 -> Sum/2, Product/1  "<R_IERA_RA_RA>"

== system UAVdesign_net/Vehicle Models/Helicopter Model/RA to IELA CG computation/RA to IELA 3 ==
  Geometry : Inport  OutDataTypeStr=Bus: GeometryParameters
  CG_RA_RA : Inport  Port=2
  Bus Selector : BusSelector  OutputSignals=R_IERA_RA_RA,alpha_IERA_IELA_IELA,m,I_IERA
  Dot Product : simulink/Math Operations/Dot Product  InputSameDT=on  OutDataType=sfix(16)  OutScaling=2^-10  DoSatur=off
  Identity matrix : Constant  Value=[1 0 0; 0 1 0; 0 0 1]
  Product : Product  RndMeth=Zero
  Product1 : Product  RndMeth=Zero
  Product2 : Product  Multiplication=Matrix(*)  RndMeth=Zero
  Product3 : Product  RndMeth=Zero
  RA to IELA1 : Subsystem
  Reshape : Reshape  OutputDimensionality=Column vector (2-D)
  Reshape1 : Reshape  OutputDimensionality=Row vector (2-D)
  Rotate to IELA : Product  Inputs=3  Multiplication=Matrix(*)  RndMeth=Zero
  Rotation Matrix from IELA to IERA : UAVdesign_net/Utilities/Axes/Euler Rotation Matrix from Earth to Body  SystemSampleTime=-1
  Sum : Sum  Inputs=-+|
  Sum1 : Sum  Inputs=+|+
  Sum2 : Sum  Inputs=|+-
  Transpose : Subsystem
      mask Display: disp('A^T', 'texmode', 'on')
  R_IELA_B_B : Outport
  alpha_IERA_IELA : Outport  Port=2
  T_IERA_IELA : Outport  Port=3
  T_IELA_IERA : Outport  Port=4
  mass_distance : Outport  Port=5
  m : Outport  Port=6
  In_CG : Outport  Port=7
  wires:
  Bus Selector/1 -> Product/1, Sum/2  "<R_IERA_RA_RA>"
  Bus Selector/2 -> alpha_IERA_IELA/1, Rotation Matrix from IELA to IERA/1  "<alpha_IERA_IELA_IELA>"
  Bus Selector/3 -> Product/2, Product1/1, m/1  "<m>"
  Sum/1 -> RA to IELA1/1(RA)
  Product1/1 -> Sum1/2
  Reshape/1 -> Product2/1
  Reshape1/1 -> Product2/2
  Dot Product/1 -> Product3/2
  Identity matrix/1 -> Product3/1
  Product3/1 -> Sum2/1
  Product2/1 -> Sum2/2
  Sum2/1 -> Product1/2
  Geometry/1 -> Bus Selector/1
  Product/1 -> mass_distance/1
  Sum1/1 -> In_CG/1
  CG_RA_RA/1 -> Sum/1
  RA to IELA1/1(IELA) -> Dot Product/1, Dot Product/2, Reshape1/1, Reshape/1, R_IELA_B_B/1
  Rotation Matrix from IELA to IERA/1 -> Transpose/1(In), T_IERA_IELA/1, Rotate to IELA/1
  Transpose/1(Out) -> T_IELA_IERA/1, Rotate to IELA/3
  Rotate to IELA/1 -> Sum1/1
  Bus Selector/4 -> Rotate to IELA/2  "<I_IERA>"
